simulink model "equilizer"  (R2017a)
settings: Solver=VariableStepAuto  StartTime=0.0  StopTime=10.0  RelTol=1e-3
undefined symbols (not defined in the file): fdesignblkfcn, gcbh
settings Model: Creator=ilyas  LastModifiedBy=ilyas

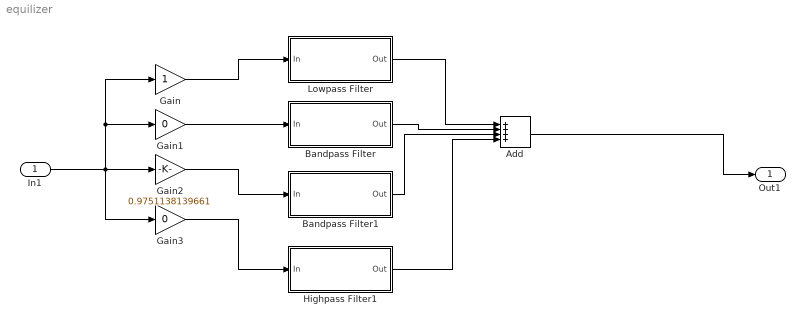
== system equilizer ==
  In1 : Inport
  Add : Sum  Inputs=++++
  Bandpass Filter : Subsystem  DialogController=fdesignblkfcn  InitFcn=fdesignblkfcn(gcbh, {'InitFcn'});  mask(Bandpass Filter){}
      mask help: Design a bandpass filter
      settings: CopyFcn=fdesignblkfcn(gcbh, {'CopyFcn'});
      mask Help: helpview(mapfilelocation('dsp'), 'dspbandpassfilter');
      mask Display: disp('Bandpass');
  Bandpass Filter1 : Subsystem  DialogController=fdesignblkfcn  InitFcn=fdesignblkfcn(gcbh, {'InitFcn'});  mask(Bandpass Filter){}
      mask help: Design a bandpass filter
      settings: CopyFcn=fdesignblkfcn(gcbh, {'CopyFcn'});
      mask Help: helpview(mapfilelocation('dsp'), 'dspbandpassfilter');
      mask Display: disp('Bandpass');
  Gain : Gain
  Gain1 : Gain  Gain=0
  Gain2 : Gain  Gain=0.9751138139661
  Gain3 : Gain  Gain=0
  Highpass Filter1 : Subsystem  DialogController=fdesignblkfcn  InitFcn=fdesignblkfcn(gcbh, {'InitFcn'});  mask(Highpass Filter){}
      mask help: Design a highpass filter
      settings: CopyFcn=fdesignblkfcn(gcbh, {'CopyFcn'});
      mask Help: helpview(mapfilelocation('dsp'), 'dsphighpassfilter');
      mask Display: disp('Highpass')
  Lowpass Filter : Subsystem  DialogController=fdesignblkfcn  InitFcn=fdesignblkfcn(gcbh, {'InitFcn'});  mask(Lowpass Filter){}
      mask help: Design a lowpass filter
      settings: CopyFcn=fdesignblkfcn(gcbh, {'CopyFcn'});
      mask Help: helpview(mapfilelocation('dsp'), 'dsplowpassfilter');
      mask Display: disp('Lowpass')
  Out1 : Outport
  wires:
  Highpass Filter1/1(Out) -> Add/4
  Gain/1 -> Lowpass Filter/1(In)
  Bandpass Filter1/1(Out) -> Add/3
  Bandpass Filter/1(Out) -> Add/2
  Gain3/1 -> Highpass Filter1/1(In)
  Add/1 -> Out1/1
  In1/1 -> Gain3/1, Gain1/1, Gain/1, Gain2/1
  Gain1/1 -> Bandpass Filter/1(In)
  Gain2/1 -> Bandpass Filter1/1(In)
  Lowpass Filter/1(Out) -> Add/1

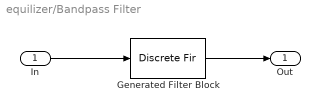
== system equilizer/Bandpass Filter ==
  In : Inport
  Generated Filter Block : DiscreteFir  Tag=BlockMethodSubSystem  Coefficients=[-0.034227365537242295 0.018312757492087928 0.05932130178861178 -0.015649458947768258 0.0096465114342621835 -0.029035785159490478 -0.015761984269044724 -0.037689628472410135 -0.03202966742034466 -0.044813544994417052 -0.042077522064569023 -0.047994018438133036 -0.044347414970127598 -0.043895492779424998 -0.036914882245408523 -0.030447360988786105 -0.019612599669352172 -0.00858331876634379 0.0047869939251154146 0.017832982590566839 0.03123510535086213 0.043139022752045862 0.053593260564708499 0.061360943995909772 0.066388263112684393 0.06800122583920179 0.066388263112684393 0.061360943995909772 0.053593260564708499 0.043139022752045862 0.03123510535086213 0.017832982590566839 0.0047869939251154146 -0.00858331876634379 -0.019612599669352172 -0.030447360988786105 -0.036914882245408523 -0.043895492779424998 -0.044347414970127598 -0.047994018438133036 -0.042077522064569023 -0.044813544994417052 -0.03202966742034466 -0.037689628472410135 -0.015761984269044724 -0.029035785159490478 0.0096465114342621835 -0.015649458947768258 0.05932130178861178 0.018312757492087928 -0.034227365537242295]  InputProcessing=Columns as channels (frame based)
  Out : Outport
  wires:
  Generated Filter Block/1 -> Out/1
  In/1 -> Generated Filter Block/1

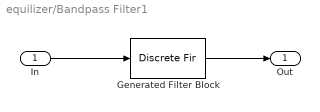
== system equilizer/Bandpass Filter1 ==
  In : Inport
  Generated Filter Block : DiscreteFir  Tag=BlockMethodSubSystem  Coefficients=[-0.071193933975794793 0.042567551632574072 0.023370929263920877 0.0067492245502078505 -0.0056303528823154706 -0.012406515894683801 -0.012509643538729659 -0.0056607808720928483 0.0073925777727120202 0.024156862094491815 0.040950617859290002 0.05303589501571479 0.05614662588295434 0.047414277531303138 0.026950275664504888 -0.0021817284297539169 -0.033973814822860146 -0.06117405180846118 -0.076560218072753941 -0.075309696327126918 -0.056281928917521193 -0.023018521202301939 0.017523864292477515 0.056264679144848485 0.083815001474115053 0.09388074499835046 0.083815001474115053 0.056264679144848485 0.017523864292477515 -0.023018521202301939 -0.056281928917521193 -0.075309696327126918 -0.076560218072753941 -0.06117405180846118 -0.033973814822860146 -0.0021817284297539169 0.026950275664504888 0.047414277531303138 0.05614662588295434 0.05303589501571479 0.040950617859290002 0.024156862094491815 0.0073925777727120202 -0.0056607808720928483 -0.012509643538729659 -0.012406515894683801 -0.0056303528823154706 0.0067492245502078505 0.023370929263920877 0.042567551632574072 -0.071193933975794793]  InputProcessing=Columns as channels (frame based)
  Out : Outport
  wires:
  Generated Filter Block/1 -> Out/1
  In/1 -> Generated Filter Block/1

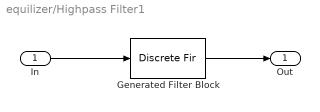
== system equilizer/Highpass Filter1 ==
  In : Inport
  Generated Filter Block : DiscreteFir  Tag=BlockMethodSubSystem  Coefficients=[0.018474008886137774 -0.07093427222798343 -0.026736009141952864 -0.012590249565781884 -0.0029223409381482746 0.0064166158658349477 0.01376997205732409 0.016707240639420411 0.013639039609664469 0.0049637238837780427 -0.0068574716590106451 -0.017827795097230564 -0.023758479772147303 -0.021504192552314477 -0.010454091224033886 0.0070581716995950124 0.025786675130562247 0.038995997151154212 0.040090951391899117 0.024873356561464898 -0.0071750444445839922 -0.052280451761689467 -0.1027024963340082 -0.14890293216856484 -0.18115471356170157 0.80737130806986068 -0.18115471356170157 -0.14890293216856484 -0.1027024963340082 -0.052280451761689467 -0.0071750444445839922 0.024873356561464898 0.040090951391899117 0.038995997151154212 0.025786675130562247 0.0070581716995950124 -0.010454091224033886 -0.021504192552314477 -0.023758479772147303 -0.017827795097230564 -0.0068574716590106451 0.0049637238837780427 0.013639039609664469 0.016707240639420411 0.01376997205732409 0.0064166158658349477 -0.0029223409381482746 -0.012590249565781884 -0.026736009141952864 -0.07093427222798343 0.018474008886137774]  InputProcessing=Columns as channels (frame based)
  Out : Outport
  wires:
  In/1 -> Generated Filter Block/1
  Generated Filter Block/1 -> Out/1

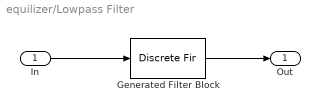
== system equilizer/Lowpass Filter ==
  In : Inport
  Generated Filter Block : DiscreteFir  Tag=BlockMethodSubSystem  Coefficients=[-0.067571599194720749 0.028366275622582534 0.024365308441611347 0.021834882196456632 0.020229321096330865 0.019593102757112429 0.019467767446300618 0.01970710174125179 0.020316328767870182 0.021189381305964993 0.022233119686554535 0.023289912862881998 0.024434404835929416 0.025590101085555161 0.026793987513412713 0.027904494200213244 0.028994063526814901 0.029963415719363243 0.030889637193174065 0.031658907557582189 0.03237246922527081 0.032938831357787801 0.033449784931778435 0.033783249602137515 0.034025406529673743 0.034071811260776463 0.034025406529673743 0.033783249602137515 0.033449784931778435 0.032938831357787801 0.03237246922527081 0.031658907557582189 0.030889637193174065 0.029963415719363243 0.028994063526814901 0.027904494200213244 0.026793987513412713 0.025590101085555161 0.024434404835929416 0.023289912862881998 0.022233119686554535 0.021189381305964993 0.020316328767870182 0.01970710174125179 0.019467767446300618 0.019593102757112429 0.020229321096330865 0.021834882196456632 0.024365308441611347 0.028366275622582534 -0.067571599194720749]  InputProcessing=Columns as channels (frame based)
  Out : Outport
  wires:
  Generated Filter Block/1 -> Out/1
  In/1 -> Generated Filter Block/1
